simulink subsystem "Estimator"  (R2022a)
settings: Solver=VariableStepAuto  StartTime=0.0  StopTime=10.0  RelTol=1e-3
values from neighbouring files (symbols this model uses):
  Iden = eye(r)    [P2D_System_main.m]    (also in P2D_System_main_sine.m; runSimulink.m = Slink.Iden)
  P_k_0 = confidence*eye(r)    [P2D_System_main.m]    (also in P2D_System_main_sine.m; runSimulink.m = Slink.P_k_0)
  Q = Q_0*eye(N.inputs)    [P2D_System_main.m]    (also in P2D_System_main_sine.m; runSimulink.m = Noise.Q)
  R = R_0*eye(N.measur)    [P2D_System_main.m]    (also in P2D_System_main_sine.m; runSimulink.m = Noise.R)
  Ts = sim_data.impl.SIM.Ts    [P2D_System_main.m]    (also in P2D_System_main_sine.m; runSimulink.m = sim_in.SIM.Ts)
  x0_est = zeros(length(A_r),1)    [P2D_System_main.m]    (also in P2D_System_main_sine.m; runSimulink.m = Slink.x0_est)
undefined symbols (not defined in the file or in its folder): A_est, B_est, C_est
settings Model: Creator=tyevans  LastModifiedBy=tyevans

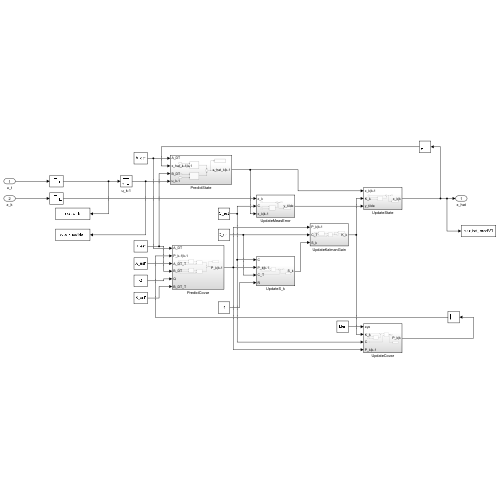
[thumbnail: Simulink's stored preview of the top-level diagram]
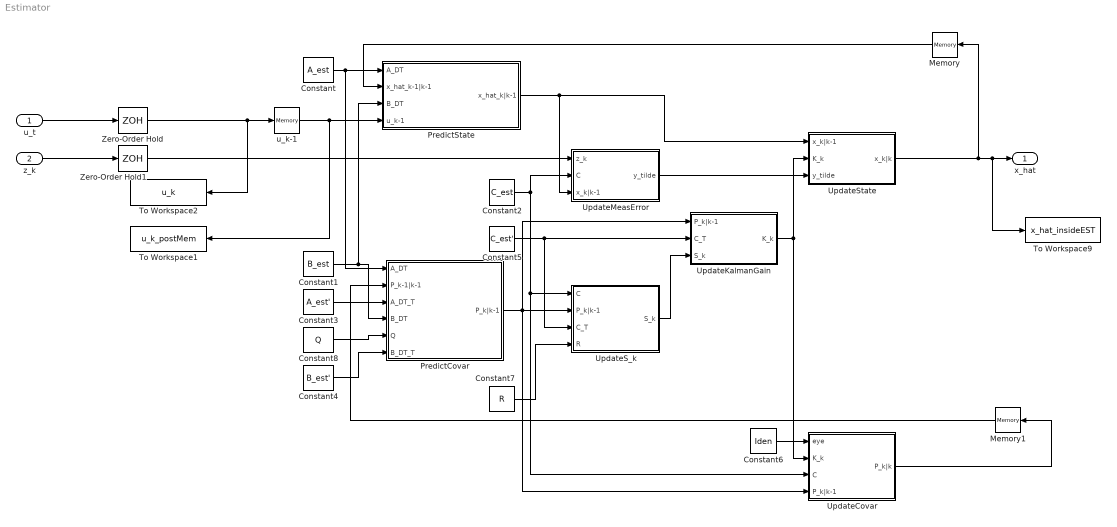
== system Estimator ==
  u_t : Inport
  z_k : Inport  Port=2
  Constant : Constant  Value=A_est  VectorParams1D=off
  Constant1 : Constant  Value=B_est  VectorParams1D=off
  Constant2 : Constant  Value=C_est  VectorParams1D=off
  Constant3 : Constant  Value=A_est'  VectorParams1D=off
  Constant4 : Constant  Value=B_est'  VectorParams1D=off
  Constant5 : Constant  Value=C_est'  VectorParams1D=off
  Constant6 : Constant  Value=Iden  VectorParams1D=off
  Constant7 : Constant  Value=R  VectorParams1D=off
  Constant8 : Constant  Value=Q  VectorParams1D=off
  Memory : Memory  InitialCondition=x0_est  InheritSampleTime=on
  Memory1 : Memory  InitialCondition=P_k_0  InheritSampleTime=on
  PredictCovar : Subsystem
  PredictState : Subsystem
  To Workspace1 : ToWorkspace  VariableName=u_k_postMem  SaveFormat=Structure With Time  SampleTime=-1
  To Workspace2 : ToWorkspace  VariableName=u_k  SaveFormat=Structure With Time  SampleTime=-1
  To Workspace9 : ToWorkspace  VariableName=x_hat_insideEST  SaveFormat=Structure With Time  SampleTime=-1
  UpdateCovar : Subsystem
  UpdateKalmanGain : Subsystem
  UpdateMeasError : Subsystem
  UpdateS_k : Subsystem
  UpdateState : Subsystem
  Zero-Order Hold : ZeroOrderHold  SampleTime=Ts
  Zero-Order Hold1 : ZeroOrderHold  SampleTime=Ts
  u_k-1 : Memory  InheritSampleTime=on
  x_hat : Outport
  wires:
  Memory/1 -> PredictState/2(x_hat_k-1|k-1)
  Memory1/1 -> PredictCovar/2(P_k-1|k-1)
  UpdateCovar/1(P_k|k) -> Memory1/1
  PredictCovar/1(P_k|k-1) -> UpdateKalmanGain/1(P_k|k-1), UpdateCovar/4(P_k|k-1), UpdateS_k/2(P_k|k-1)
  Constant2/1 -> UpdateMeasError/2(C), UpdateCovar/3(C), UpdateS_k/1(C)
  Constant/1 -> PredictCovar/1(A_DT), PredictState/1(A_DT)
  PredictState/1(x_hat_k|k-1) -> UpdateState/1(x_k|k-1), UpdateMeasError/3(x_k|k-1)
  UpdateS_k/1(S_k) -> UpdateKalmanGain/3(S_k)
  Constant3/1 -> PredictCovar/3(A_DT_T)
  Constant8/1 -> PredictCovar/5(Q)
  Constant4/1 -> PredictCovar/6(B_DT_T)
  UpdateState/1(x_k|k) -> x_hat/1, To Workspace9/1, Memory/1
  Constant1/1 -> PredictCovar/4(B_DT), PredictState/3(B_DT)
  Constant5/1 -> UpdateKalmanGain/2(C_T), UpdateS_k/3(C_T)
  Constant7/1 -> UpdateS_k/4(R)
  UpdateKalmanGain/1(K_k) -> UpdateCovar/2(K_k), UpdateState/2(K_k)
  Constant6/1 -> UpdateCovar/1(eye)
  z_k/1 -> Zero-Order Hold1/1
  UpdateMeasError/1(y_tilde) -> UpdateState/3(y_tilde)
  u_k-1/1 -> PredictState/4(u_k-1), To Workspace1/1
  u_t/1 -> Zero-Order Hold/1
  Zero-Order Hold/1 -> To Workspace2/1, u_k-1/1
  Zero-Order Hold1/1 -> UpdateMeasError/1(z_k)

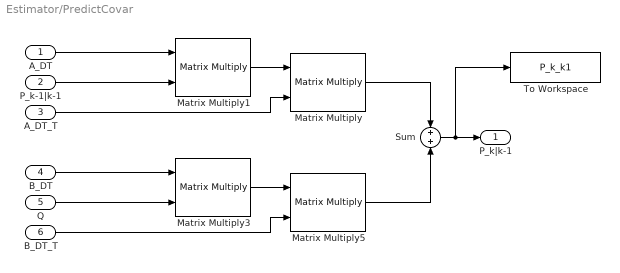
== system Estimator/PredictCovar ==
  A_DT : Inport
  P_k-1|k-1 : Inport  Port=2
  A_DT_T : Inport  Port=3
  B_DT : Inport  Port=4
  Q : Inport  Port=5
  B_DT_T : Inport  Port=6
  Matrix Multiply{,1,3,5} (4 alike) : Product  Multiplication=Matrix(*)
  Sum : Sum
  To Workspace : ToWorkspace  VariableName=P_k_k1  SaveFormat=Structure With Time  SampleTime=-1
  P_k|k-1 : Outport
  wires:
  Matrix Multiply5/1 -> Sum/2
  Matrix Multiply/1 -> Sum/1
  Matrix Multiply3/1 -> Matrix Multiply5/1
  B_DT_T/1 -> Matrix Multiply5/2
  Q/1 -> Matrix Multiply3/2
  B_DT/1 -> Matrix Multiply3/1
  Matrix Multiply1/1 -> Matrix Multiply/1
  A_DT_T/1 -> Matrix Multiply/2
  P_k-1|k-1/1 -> Matrix Multiply1/2
  A_DT/1 -> Matrix Multiply1/1
  Sum/1 -> P_k|k-1/1, To Workspace/1

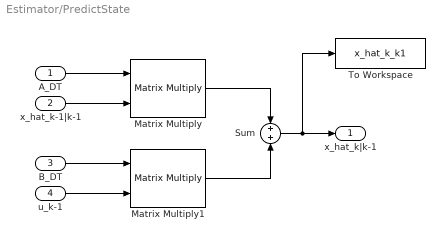
== system Estimator/PredictState ==
  A_DT : Inport
  x_hat_k-1|k-1 : Inport  Port=2
  B_DT : Inport  Port=3
  u_k-1 : Inport  Port=4
  Matrix Multiply : Product  Multiplication=Matrix(*)
  Matrix Multiply1 : Product  Multiplication=Matrix(*)
  Sum : Sum
  To Workspace : ToWorkspace  VariableName=x_hat_k_k1  SaveFormat=Structure With Time  SampleTime=-1
  x_hat_k|k-1 : Outport
  wires:
  Sum/1 -> x_hat_k|k-1/1, To Workspace/1
  Matrix Multiply1/1 -> Sum/2
  Matrix Multiply/1 -> Sum/1
  u_k-1/1 -> Matrix Multiply1/2
  B_DT/1 -> Matrix Multiply1/1
  x_hat_k-1|k-1/1 -> Matrix Multiply/2
  A_DT/1 -> Matrix Multiply/1

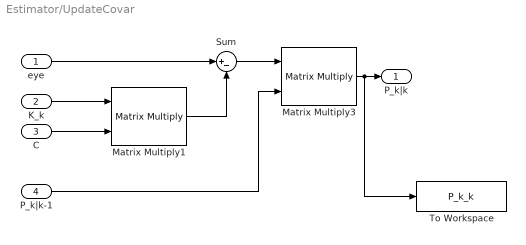
== system Estimator/UpdateCovar ==
  eye : Inport
  K_k : Inport  Port=2
  C : Inport  Port=3
  P_k|k-1 : Inport  Port=4
  Matrix Multiply1 : Product  Multiplication=Matrix(*)
  Matrix Multiply3 : Product  Multiplication=Matrix(*)
  Sum : Sum  Inputs=|+-
  To Workspace : ToWorkspace  VariableName=P_k_k  SaveFormat=Structure With Time  SampleTime=-1
  P_k|k : Outport
  wires:
  Sum/1 -> Matrix Multiply3/1
  Matrix Multiply1/1 -> Sum/2
  eye/1 -> Sum/1
  P_k|k-1/1 -> Matrix Multiply3/2
  Matrix Multiply3/1 -> P_k|k/1, To Workspace/1
  C/1 -> Matrix Multiply1/2
  K_k/1 -> Matrix Multiply1/1

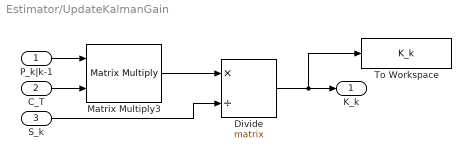
== system Estimator/UpdateKalmanGain ==
  P_k|k-1 : Inport
  C_T : Inport  Port=2
  S_k : Inport  Port=3
  Divide : Product  Inputs=*/  Multiplication=Matrix(*)
  Matrix Multiply3 : Product  Multiplication=Matrix(*)
  To Workspace : ToWorkspace  VariableName=K_k  SaveFormat=Structure With Time  SampleTime=-1
  K_k : Outport
  wires:
  S_k/1 -> Divide/2
  C_T/1 -> Matrix Multiply3/2
  P_k|k-1/1 -> Matrix Multiply3/1
  Divide/1 -> K_k/1, To Workspace/1
  Matrix Multiply3/1 -> Divide/1

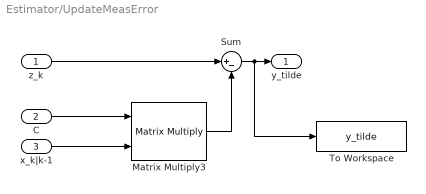
== system Estimator/UpdateMeasError ==
  z_k : Inport
  C : Inport  Port=2
  x_k|k-1 : Inport  Port=3
  Matrix Multiply3 : Product  Multiplication=Matrix(*)
  Sum : Sum  Inputs=|+-
  To Workspace : ToWorkspace  VariableName=y_tilde  SaveFormat=Structure With Time  SampleTime=-1
  y_tilde : Outport
  wires:
  C/1 -> Matrix Multiply3/1
  x_k|k-1/1 -> Matrix Multiply3/2
  z_k/1 -> Sum/1
  Sum/1 -> y_tilde/1, To Workspace/1
  Matrix Multiply3/1 -> Sum/2

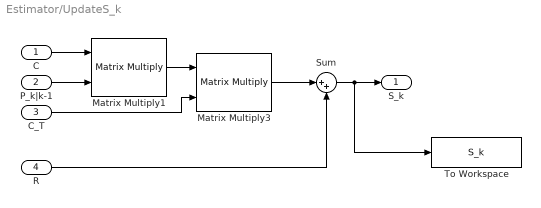
== system Estimator/UpdateS_k ==
  C : Inport
  P_k|k-1 : Inport  Port=2
  C_T : Inport  Port=3
  R : Inport  Port=4
  Matrix Multiply1 : Product  Multiplication=Matrix(*)
  Matrix Multiply3 : Product  Multiplication=Matrix(*)
  Sum : Sum  Inputs=|++
  To Workspace : ToWorkspace  VariableName=S_k  SaveFormat=Structure With Time  SampleTime=-1
  S_k : Outport
  wires:
  R/1 -> Sum/2
  C_T/1 -> Matrix Multiply3/2
  P_k|k-1/1 -> Matrix Multiply1/2
  C/1 -> Matrix Multiply1/1
  Sum/1 -> S_k/1, To Workspace/1
  Matrix Multiply3/1 -> Sum/1
  Matrix Multiply1/1 -> Matrix Multiply3/1

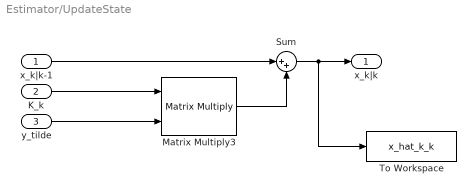
== system Estimator/UpdateState ==
  x_k|k-1 : Inport
  K_k : Inport  Port=2
  y_tilde : Inport  Port=3
  Matrix Multiply3 : Product  Multiplication=Matrix(*)
  Sum : Sum  Inputs=|++
  To Workspace : ToWorkspace  VariableName=x_hat_k_k  SaveFormat=Structure With Time  SampleTime=-1
  x_k|k : Outport
  wires:
  Sum/1 -> x_k|k/1, To Workspace/1
  Matrix Multiply3/1 -> Sum/2
  x_k|k-1/1 -> Sum/1
  y_tilde/1 -> Matrix Multiply3/2
  K_k/1 -> Matrix Multiply3/1
